simulink model "untitled"  (R2021a)
settings: Solver=VariableStepAuto  StartTime=0.0  StopTime=inf  RelTol=1e-3
undefined symbols (not defined in the file): Standard_Devices, UDP_Protocol
libraries: sldrtlib x1
settings Model: Creator=HP OMEN  LastModifiedBy=HP OMEN

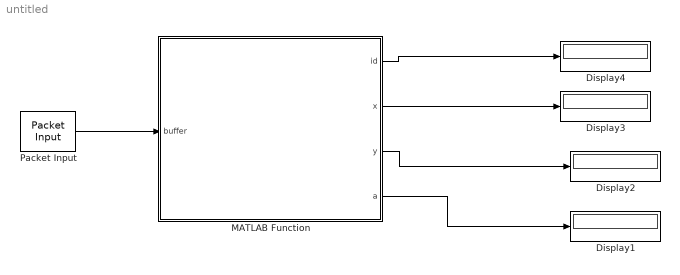
== system untitled ==
  Display{1..4} (4 alike) : Display
  MATLAB Function : MATLAB Function  TreatAsAtomicUnit=on
  Packet Input : sldrtlib/Packet Input  SampleTime=0.1  MaxMissedTicks=10  ShowMissedTicks=off  YieldWhenWaiting=off  DrvName=Standard_Devices/UDP_Protocol  DrvAddress=58624  DrvOptions=[0 16385 0 0 0 0 0 0 0 0 0 0 0 0 0 0 0 0 0 0 0 0 0 0 0 0 0 0 0 0 0 0 0 0 0 0 0 0 0 0 0 0 0 0 0 0 0 0 0 0 0 0 0 0 0 0 0 0 0 0 0 0 0 0 0 0 0 0 0 0 0 0 0 0 0 0 0 0 0 0 0 0 0 0 0 0 0 0 0 0 0 0 0 0 0 0 0 0 0 0 0 0 0 0 0 0 0 0 0 0 0 0 0 0 0 0 0 0 0 0 0 0 0 0 0 0 0 0 0 0 0 0 0 0 0 0 0 0 0 0 0 0 0 0 0 0 0 0 0 0 0 0 0 0 0 0 0 0 0 0 0 0 0 0 0 0 0 0 0 0 0 0 0 0 0 0 0 0 0 0 0 0 0 0 0 0 0 0 0 0 0 0 0 0 0 0 0 0 0 0 0 0 0 0 0 0 0 0 0 0 0 0 0 0 0 0 0 0 0 0 0 0 0 0 0 0 0 0 0 0 0 0 0 0 0 0 0 0 0 0 0 0 0 0 0 0 0 0 0 0 0 0 0 0 0 0]  PacketSize=35  DataTypes='35*int8'  ShowReady=off  ShowError=off  PacketID=1  ByteOrder=1  ShowTimestamp=off
      settings: AttributesFormatString=UDP Protocol [58624]
  wires:
  MATLAB Function/4(a) -> Display1/1
  MATLAB Function/3(y) -> Display2/1
  MATLAB Function/2(x) -> Display3/1
  Packet Input/1 -> MATLAB Function/1(buffer)
  MATLAB Function/1(id) -> Display4/1

== matlab function untitled/MATLAB Function ==
  data: id output; x output; y output; a output; buffer input
function [id,x,y,a] = ObtenerDatos(buffer) 
    
    indice = 77; inicio = 0; fin = 0; count = 1; 
    A=[0 0 0 0];     p = 0.0;   aux=0; potencia = 1;

    for i = 1:length(buffer)
        if(buffer(i) == indice)
           if(inicio == 0 && fin == 0)
                inicio = i;
            elseif(inicio ~= 0 && fin == 0)
                fin = i;
                break;
            end
        end
    end

    if(inicio ~= 0 && fin ~= 0)   
        
        for i = (inicio+1):(fin - 1) 
            
            if(buffer(i) == 46)
                    aux = 1;
            elseif(buffer(i) ~= 78 && i ~= fin - 1)  
                 
                 if( aux == 0)
                    p = (p*10) + int8ToDouble(buffer(i));
                 elseif( aux == 1)
                    p = p + (int8ToDouble(buffer(i))/(10^potencia));
                    potencia = potencia + 1;
                 end  
            elseif( buffer(i) == 78 || i == fin - 1)
                if(i == fin - 1)
                   p = p + (int8ToDouble(buffer(i))/(10^potencia));
                end
                A(count) = p;
                p = 0.0;
                aux=0;
                potencia = 1;
                count = count + 1;
            end 
        end 
    end
    
    id = A(1) ;
    x = A(2) ;
    y = A(3) ;
    a = A(4) ;
end


function out = int8ToDouble(in)
    switch in
        case 48
            out = 0.0;
        case 49
            out = 1.0;
        case 50
            out = 2.0;
        case 51
            out = 3.0;
        case 52
            out = 4.0;
        case 53
            out = 5.0;
        case 54
            out = 6.0;
        case 55
            out = 7.0;
        case 56
            out = 8.0;
        case 57
            out = 9.0;
        otherwise
            out = 0.0;
    end
end
